simulink model "Robot_diferencial_control"  (R2017b)
settings: Solver=VariableStepAuto  StartTime=0.0  StopTime=Tsim  MaxStep=1e-2  MinStep=1e-5  RelTol=1e-3
values from neighbouring files (symbols this model uses):
  CI = [0 0 0]    [graf.m]
  xref = in(1)    [Generador_de_trayectorias.m]    (also in graf.m = 3)
  yref = in(2)    [Generador_de_trayectorias.m]    (also in graf.m = 4)
settings Model: Creator=Raúl  LastModifiedBy=fevaf

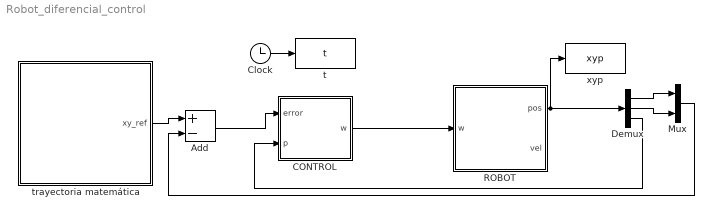
== system Robot_diferencial_control ==
  Add : Sum  Inputs=+-
  CONTROL : Subsystem
  Clock : Clock
  Demux : Demux  Outputs=3
  Mux : Mux  Inputs=2
  ROBOT : Subsystem
  t : ToWorkspace  VariableName=t  SampleTime=-1
  trayectoria matemática : Subsystem
  xyp : ToWorkspace  VariableName=xyp  SampleTime=-1
  wires:
  Clock/1 -> t/1
  CONTROL/1(w) -> ROBOT/1(w)
  trayectoria matemática/1(xy_ref) -> Add/1
  Add/1 -> CONTROL/1(error)
  ROBOT/1(pos) -> xyp/1, Demux/1
  Demux/1 -> Mux/1
  Demux/2 -> Mux/2
  Mux/1 -> Add/2
  Demux/3 -> CONTROL/2(p)

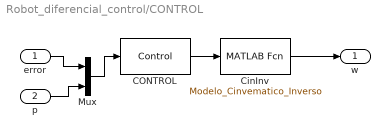
== system Robot_diferencial_control/CONTROL ==
  error : Inport
  p : Inport  Port=2
  CONTROL : MATLABFcn  MATLABFcn=Control
  CinInv : MATLABFcn  MATLABFcn=Modelo_Cinvematico_Inverso
  Mux : Mux  Inputs=2
  w : Outport
  wires:
  CinInv/1 -> w/1
  CONTROL/1 -> CinInv/1
  Mux/1 -> CONTROL/1
  error/1 -> Mux/1
  p/1 -> Mux/2

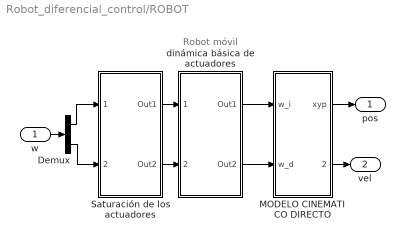
== system Robot_diferencial_control/ROBOT ==
  note: Robot móvil
  w : Inport
  Demux : Demux  Outputs=2
  MODELO CINEMATICO DIRECTO : Subsystem
  Saturación de los actuadores : Subsystem
  dinámica básica de actuadores : Subsystem
  pos : Outport
  vel : Outport  Port=2
  wires:
  Saturación de los actuadores/2(Out2) -> dinámica básica de actuadores/2(w_d_ref)
  Saturación de los actuadores/1(Out1) -> dinámica básica de actuadores/1(w_i_ref)
  dinámica básica de actuadores/2(Out2) -> MODELO CINEMATICO DIRECTO/2(w_d)
  dinámica básica de actuadores/1(Out1) -> MODELO CINEMATICO DIRECTO/1(w_i)
  Demux/1 -> Saturación de los actuadores/1(w_i_ref)
  Demux/2 -> Saturación de los actuadores/2(w_d_ref)
  MODELO CINEMATICO DIRECTO/1(xyp) -> pos/1
  MODELO CINEMATICO DIRECTO/2(xyp_d) -> vel/1
  w/1 -> Demux/1

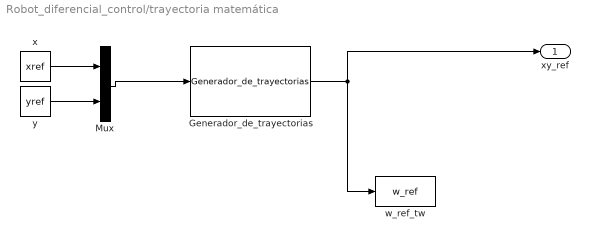
== system Robot_diferencial_control/trayectoria matemática ==
  Generador_de_trayectorias : MATLABFcn  MATLABFcn=Generador_de_trayectorias
  Mux : Mux  Inputs=2
  w_ref_tw : ToWorkspace  VariableName=w_ref  SampleTime=-1
  x : Constant  Value=xref
  y : Constant  Value=yref
  xy_ref : Outport
  wires:
  Generador_de_trayectorias/1 -> xy_ref/1, w_ref_tw/1
  Mux/1 -> Generador_de_trayectorias/1
  x/1 -> Mux/1
  y/1 -> Mux/2

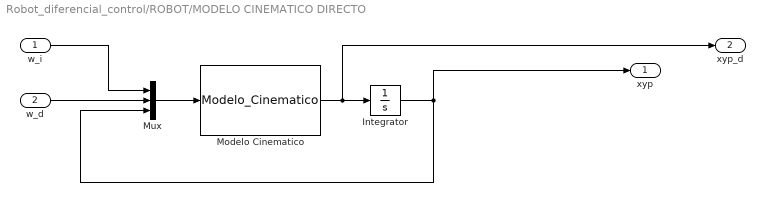
== system Robot_diferencial_control/ROBOT/MODELO CINEMATICO DIRECTO ==
  w_i : Inport
  w_d : Inport  Port=2
  Integrator : Integrator  InitialCondition=CI
  "Modelo Cinematico " : MATLABFcn  MATLABFcn=Modelo_Cinematico
  Mux : Mux  Inputs=3
  xyp : Outport
  xyp_d : Outport  Port=2
  wires:
  "Modelo Cinematico "/1 -> xyp_d/1, Integrator/1
  w_i/1 -> Mux/1
  Integrator/1 -> xyp/1, Mux/3
  Mux/1 -> "Modelo Cinematico "/1
  w_d/1 -> Mux/2

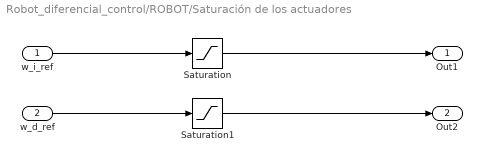
== system Robot_diferencial_control/ROBOT/Saturación de los actuadores ==
  w_i_ref : Inport
  w_d_ref : Inport  Port=2
  Saturation : Saturate  UpperLimit=2.5  LowerLimit=-2.5
  Saturation1 : Saturate  UpperLimit=2.5  LowerLimit=-2.5
  Out1 : Outport
  Out2 : Outport  Port=2
  wires:
  w_i_ref/1 -> Saturation/1
  Saturation/1 -> Out1/1
  w_d_ref/1 -> Saturation1/1
  Saturation1/1 -> Out2/1

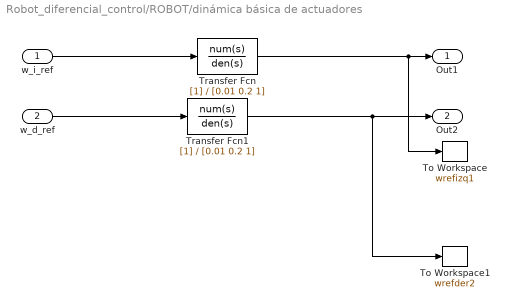
== system Robot_diferencial_control/ROBOT/dinámica básica de actuadores ==
  w_i_ref : Inport
  w_d_ref : Inport  Port=2
  To Workspace : ToWorkspace  VariableName=wrefizq1  SampleTime=-1
  To Workspace1 : ToWorkspace  VariableName=wrefder2  SampleTime=-1
  Transfer Fcn : TransferFcn  Denominator=[0.01 0.2 1]
  Transfer Fcn1 : TransferFcn  Denominator=[0.01 0.2 1]
  Out1 : Outport
  Out2 : Outport  Port=2
  wires:
  w_i_ref/1 -> Transfer Fcn/1
  Transfer Fcn/1 -> To Workspace/1, Out1/1
  w_d_ref/1 -> Transfer Fcn1/1
  Transfer Fcn1/1 -> To Workspace1/1, Out2/1
